simulink model "sl_drivepoint"  (R2015a)
settings: Solver=ode45  StartTime=0.0  StopTime=Inf  RelTol=1e-3
InitFcn:
  | if exist('x0')
  |   assert(length(x0)==3, 'x0 must be a 3 vector');
  | else
  |   x0 = [5 5 0];
  |   msgbox(sprintf('x0 not defined in workspace, setting it to [%g %g %g]\n', x0));
  | end
  | if exist('xg')
  |   assert(length(xg)==2, 'xg must be a 2 vector');
  | else
  |   xg = [0 0];
  |   msgbox(sprintf('xg not defined in workspace, setting it to [%g %g]\n', xg));
  | end
  | % clean up old vehicle icons
  | set(0, 'ShowHiddenHandles', 'on')
  | delete(findobj('Tag', 'vehicle'))
  | set(0, 'ShowHiddenHandles', 'off')
  | clear out
StopFcn:
  | % update the XY scope
  | if exist('out')
  |  % come here if running interactively, the output variable has been
  |  % saved to the workspace
  |   set(0, 'ShowHiddenHandles', 'on')
  |   fig = findobj('name', 'XY');
  |   ax = findobj(fig, 'type', 'axes');
  |   axes(ax);
  |   grid on
  |   hold on
  |   plot_vehicle(x0, 'r', 'Tag', 'vehicle')
  |   plot_vehicle(out.y(end,:), 'b', 'Tag', 'vehicle')
  |   hold off
  |   set(0, 'ShowHiddenHandles', 'off')
  | end
libraries: roblocks x2, simulink x2
settings Model: Creator=pic  LastModifiedBy=corkep
settings DataIOCC: LimitDataPoints=off  ReturnWorkspaceOutputs=on  TimeSaveName=t  OutputSaveName=y
settings OptimizationCC: ExpressionDepthLimit=2147483647
settings DebuggingCC: UnderspecifiedInitializationDetection=Classic  MergeDetectMultiDrivingBlocksExec=none  StateNameClashWarn=warning
settings GRTTargetCC: CombineOutputUpdateFcns=off  GRTInterface=on

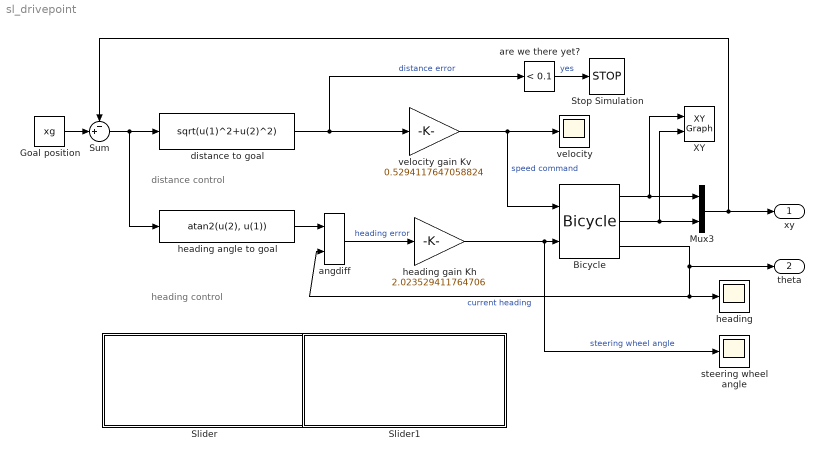
== system sl_drivepoint ==
  note: distance control
  note: heading control
  Bicycle : roblocks/Vehicles/Bicycle  vlim=1  accel=1  alim=1  steer_rate=Inf  L=1  x0=x0
  Goal position : Constant  Value=xg
  Mux3 : Mux  Inputs=2
  Slider : Subsystem  Description=Replaced Block  mask(Replaced Block){}
      mask help: This block has been replaced with an empty subsystem because it used functionality that is unavailable in Simulink R2015a.
      mask Display: fprintf('Replaced: %s\n','Dashboard Widget')
  Slider1 : Subsystem  Description=Replaced Block  mask(Replaced Block){}
      mask help: This block has been replaced with an empty subsystem because it used functionality that is unavailable in Simulink R2015a.
      mask Display: fprintf('Replaced: %s\n','Dashboard Widget')
  Stop Simulation : Stop
  Sum : Sum  Inputs=-+|
  XY : simulink/Sinks/XY Graph  xmin=-6  xmax=6  ymin=-6  ymax=6  st=-1
  angdiff : roblocks/Toolbox/angdiff
  are we there yet? : simulink/Logic and Bit Operations/Compare To Constant  relop=<  const=0.1  OutDataTypeStr=boolean
  distance to goal : Fcn  Expr=sqrt(u(1)^2+u(2)^2)
  heading : Scope
      settings: TimeRange=auto  LimitDataPoints=on  MaxDataPoints=5000  SaveToWorkspace=off  SaveName=ScopeData2  YMin=-2.86457  YMax=0.31829  SampleTime=-1
  heading angle to goal : Fcn  Expr=atan2(u(2), u(1))
  heading gain Kh : Gain  Gain=2.023529411764706
  steering wheel angle : Scope
      settings: TimeRange=auto  LimitDataPoints=on  MaxDataPoints=5000  SaveToWorkspace=off  YMin=-5.3638  YMax=0.59595  SampleTime=-1
  velocity : Scope
      settings: TimeRange=auto  MaxDataPoints=5000  SaveToWorkspace=off  YMin=-0.42175  YMax=4.32515  SampleTime=-1
  velocity gain Kv : Gain  Gain=0.5294117647058824
  xy : Outport
  "theta " : Outport  Port=2
  wires:
  Bicycle/1 -> Mux3/1, XY/1
  Bicycle/2 -> Mux3/2, XY/2
  Mux3/1 -> xy/1, Sum/1
  Sum/1 -> distance to goal/1, heading angle to goal/1
  distance to goal/1 -> velocity gain Kv/1, are we there yet?/1  "distance error"
  heading angle to goal/1 -> angdiff/1
  Bicycle/3 -> heading/1, angdiff/2, "theta "/1  "current heading"
  angdiff/1 -> heading gain Kh/1  "heading error"
  velocity gain Kv/1 -> Bicycle/1, velocity/1  "speed command"
  Goal position/1 -> Sum/2
  heading gain Kh/1 -> steering wheel angle/1, Bicycle/2  "steering wheel angle"
  are we there yet?/1 -> Stop Simulation/1  "yes"

== system sl_drivepoint/Slider ==

== system sl_drivepoint/Slider1 ==
